simulink model "Copy_of_DSBF"  (R2019b)
settings: Solver=FixedStepDiscrete  StartTime=0.0  StopTime=stopTime  RelTol=1e-3
InitFcn:
  | initCallback
StopFcn:
  | stopCallback
values from neighbouring files (symbols this model uses):
  arraySize = mp.arraySize    [modelparameters.m]
  arraySpacing = mp.arraySpacing    [modelparameters.m]
  delayDataTypeFractionLength = mp.fractionalDelayAddrSize    [modelparameters.m]
  delayDataTypeWordLength = mp.integerDelayAddrSize + mp.fractionalDelayAddrSize    [modelparameters.m]
  mp = sm_init_avalon_signals(mp)    [sm_callback_init.m]    (also in sm_callback_stop.m = sm_stop_verify(mp))
  samplingRate = mp.samplingRate    [modelparameters.m]
  speedOfSound = mp.speedOfSound    [modelparameters.m]
  upsampleFactor = mp.upsampleFactor    [modelparameters.m]
undefined symbols (not defined in the file or in its folder): delayDataTypeSign
libraries: simulink x6, hdlsllib x4, dspsigops x2, dspmlti4 x1, dsphdlfiltering x1
settings Model: Creator=Ross  LastModifiedBy=wickh
settings SolverCC: MinimalZcImpactIntegration=on
settings DataIOCC: ReturnWorkspaceOutputs=off
settings OptimizationCC: DefaultParameterBehavior=Inlined  SimCompilerOptimization=on
settings DebuggingCC: ReadBeforeWriteMsg=DisableAll  WriteAfterWriteMsg=DisableAll  WriteAfterReadMsg=DisableAll  AlgebraicLoopMsg=error  SingleTaskRateTransMsg=error  PregeneratedLibrarySubsystemCodeDiagnostic=none  ArithmeticOperatorsInVariantConditions=warning
settings HardwareCC: ProdBitPerPointer=32  ProdBitPerSizeT=32  ProdBitPerPtrDiffT=32  ProdLargestAtomicFloat=None  ProdIntDivRoundTo=Undefined  ProdEndianess=Unspecified  ProdWordSize=32  ProdHWDeviceType=ASIC/FPGA->ASIC/FPGA  TargetBitPerPointer=64  TargetBitPerSizeT=64  TargetBitPerPtrDiffT=64  TargetLongLongMode=on  TargetIntDivRoundTo=Zero  TargetEndianess=LittleEndian  TargetWordSize=64  TargetHWDeviceType=Custom Processor->MATLAB Host Computer  ProdEqTarget=off
settings ModelReferenceCC: UpdateModelReferenceTargets=IfOutOfDate
settings SFSimCC: SFSimEcho=off  SimUseLocalCustomCode=off  CustomCodeUndefinedFunction=UseInterfaceOnly
settings RTWCC: RTWUseLocalCustomCode=off

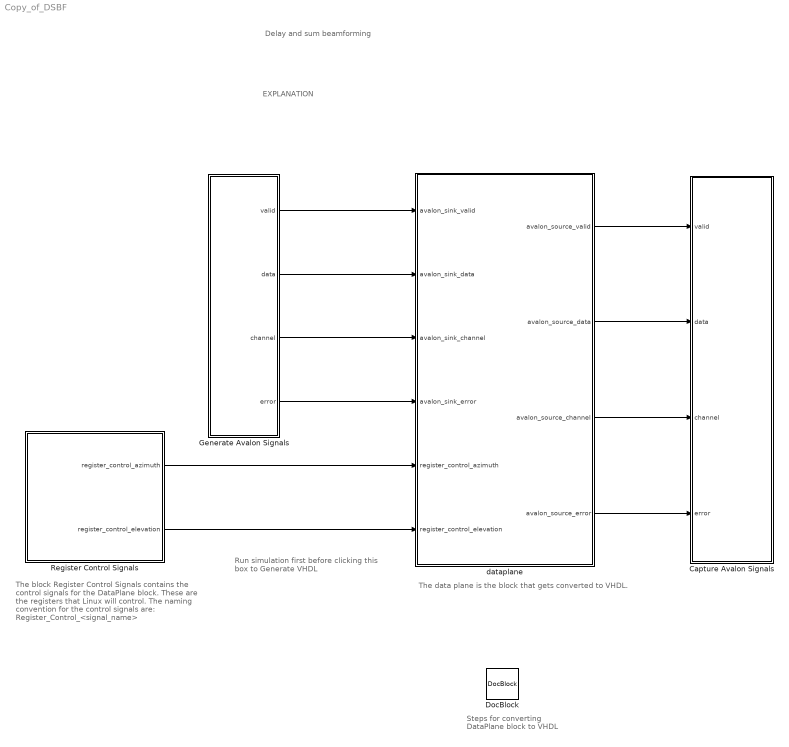
== system Copy_of_DSBF ==
  note: The data plane is the block that gets converted to VHDL.
  note: EXPLANATION
  note: Steps for converting
      | DataPlane block
      | to VHDL
  note: Delay and sum beamforming
  note: Run simulation first
      | before clicking this box to
      | Generate VHDL
  note: The block Register Control Signals contains
      | the control signals for the DataPlane block.
      | These are the registers that Linux will control.
      | The naming convention for the control
      | signals are:  Register_Control_<signal_name>
  Capture Avalon Signals : Subsystem
  DocBlock : simulink/Model-Wide Utilities/DocBlock  DocumentType=HTML
  Generate Avalon Signals : Subsystem
  Register Control Signals : Subsystem
  dataplane : Subsystem  TreatAsAtomicUnit=on
  wires:
  Generate Avalon Signals/2(data) -> dataplane/2(avalon_sink_data)
  Generate Avalon Signals/1(valid) -> dataplane/1(avalon_sink_valid)
  Generate Avalon Signals/3(channel) -> dataplane/3(avalon_sink_channel)
  Generate Avalon Signals/4(error) -> dataplane/4(avalon_sink_error)
  dataplane/2(avalon_source_data) -> Capture Avalon Signals/2(data)
  dataplane/1(avalon_source_valid) -> Capture Avalon Signals/1(valid)
  dataplane/3(avalon_source_channel) -> Capture Avalon Signals/3(channel)
  dataplane/4(avalon_source_error) -> Capture Avalon Signals/4(error)
  Register Control Signals/1(register_control_azimuth) -> dataplane/5(register_control_azimuth)
  Register Control Signals/2(register_control_elevation) -> dataplane/6(register_control_elevation)

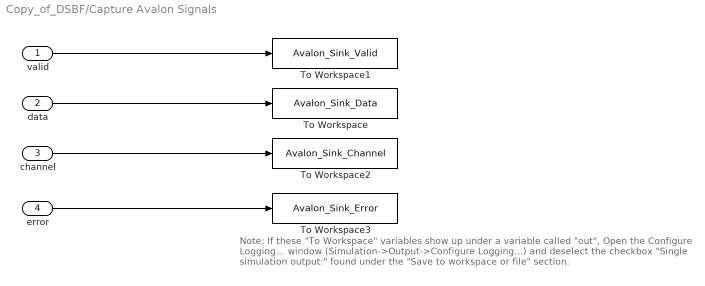
== system Copy_of_DSBF/Capture Avalon Signals ==
  note: Note:  If these "To Workspace" variables show up under a variable called "out",
      | Open the Configure Logging... window (Simulation->Output->Configure Logging...)
      | and deselect the checkbox "Single simulation output:" found under the "Save to workspace or file" section.
  valid : Inport
  data : Inport  Port=2
  channel : Inport  Port=3
  error : Inport  Port=4
  To Workspace : ToWorkspace  VariableName=Avalon_Sink_Data  SaveFormat=Timeseries  SampleTime=-1
  To Workspace1 : ToWorkspace  VariableName=Avalon_Sink_Valid  SaveFormat=Timeseries  SampleTime=-1
  To Workspace2 : ToWorkspace  VariableName=Avalon_Sink_Channel  SaveFormat=Timeseries  SampleTime=-1
  To Workspace3 : ToWorkspace  VariableName=Avalon_Sink_Error  SaveFormat=Timeseries  SampleTime=-1
  wires:
  data/1 -> To Workspace/1
  valid/1 -> To Workspace1/1
  error/1 -> To Workspace3/1
  channel/1 -> To Workspace2/1

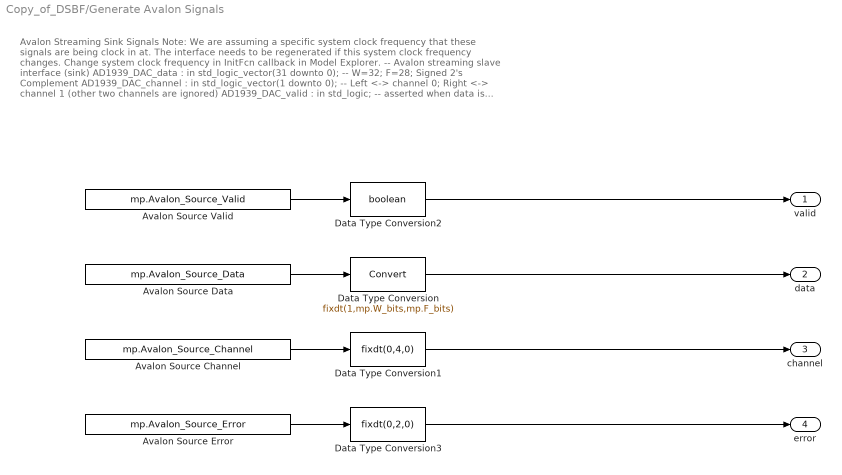
== system Copy_of_DSBF/Generate Avalon Signals ==
  note: Avalon Streaming Sink Signals
      | Note: We are assuming a specific system clock frequency that these signals are being clock in at.
      | The interface needs to be regenerated if this system clock frequency changes. Change system clock frequency in InitFcn callback in Model Explorer.
      |
      | -- Avalon streaming slave interface (sink)
      | AD1939_DAC_data : in std_logic_vector(31 downto 0); -- W=32; F=28; Signed 2's Complement
      | AD1939_DAC_channel : in std_logic_vector(1 downto 0); -- Left <-> channel 0; Right <-> channel 1 (other two channels are ignored)
      | AD1939_DAC_valid : in std_logic; -- asserted when data is valid
      | AD1939_DAC_error : in std_logic_vector(1 downto 0) -- error channel is ignored, assumed to be error free at this point
      |
      | For more information on the data-channel-valid protocol, see chapter 5 in Intel's Avalon Interfaced Specification (p. 40) at https://www.intel.com/content/dam/www/programmable/us/en/pdfs/literature/manual/mnl_avalon_spec.pdf
  Avalon Source Channel : FromWorkspace  VariableName=mp.Avalon_Source_Channel  OutDataTypeStr=double  SampleTime=mp.Ts_sim
  "Avalon Source Data " : FromWorkspace  VariableName=mp.Avalon_Source_Data  OutDataTypeStr=double  SampleTime=mp.Ts_sim
  Avalon Source Error : FromWorkspace  VariableName=mp.Avalon_Source_Error  OutDataTypeStr=double  SampleTime=mp.Ts_sim
  Avalon Source Valid : FromWorkspace  VariableName=mp.Avalon_Source_Valid  OutDataTypeStr=double  SampleTime=mp.Ts_sim
  Data Type Conversion : DataTypeConversion  OutDataTypeStr=fixdt(1,mp.W_bits,mp.F_bits)
  Data Type Conversion1 : DataTypeConversion  OutDataTypeStr=fixdt(0,4,0)
  Data Type Conversion2 : DataTypeConversion  OutDataTypeStr=boolean
  Data Type Conversion3 : DataTypeConversion  OutDataTypeStr=fixdt(0,2,0)
  valid : Outport  VectorParamsAs1DForOutWhenUnconnected=off
  data : Outport  Port=2  VectorParamsAs1DForOutWhenUnconnected=off
  channel : Outport  Port=3  VectorParamsAs1DForOutWhenUnconnected=off
  error : Outport  Port=4  VectorParamsAs1DForOutWhenUnconnected=off
  wires:
  Data Type Conversion1/1 -> channel/1
  Data Type Conversion2/1 -> valid/1
  Avalon Source Error/1 -> Data Type Conversion3/1
  Data Type Conversion/1 -> data/1
  Avalon Source Valid/1 -> Data Type Conversion2/1
  Data Type Conversion3/1 -> error/1
  Avalon Source Channel/1 -> Data Type Conversion1/1
  "Avalon Source Data "/1 -> Data Type Conversion/1

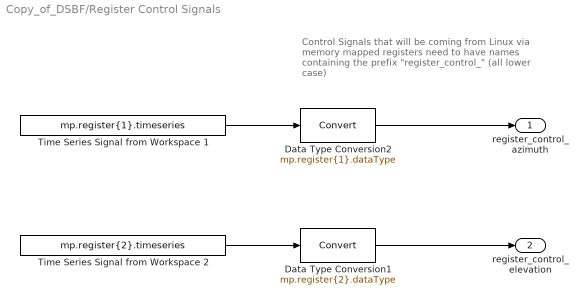
== system Copy_of_DSBF/Register Control Signals ==
  note: Control Signals that will be coming from Linux via
      | memory mapped registers need to have names
      | containing the prefix "register_control_"
      | (all lower case)
  Data Type Conversion1 : DataTypeConversion  OutDataTypeStr=mp.register{2}.dataType
  Data Type Conversion2 : DataTypeConversion  OutDataTypeStr=mp.register{1}.dataType
  Time Series Signal from Workspace 1 : FromWorkspace  VariableName=mp.register{1}.timeseries  OutDataTypeStr=double  SampleTime=mp.Ts_sim
  Time Series Signal from Workspace 2 : FromWorkspace  VariableName=mp.register{2}.timeseries  OutDataTypeStr=double  SampleTime=mp.Ts_sim
  register_control_azimuth : Outport  VectorParamsAs1DForOutWhenUnconnected=off
  register_control_elevation : Outport  Port=2  VectorParamsAs1DForOutWhenUnconnected=off
  wires:
  Time Series Signal from Workspace 1/1 -> Data Type Conversion2/1
  Time Series Signal from Workspace 2/1 -> Data Type Conversion1/1
  Data Type Conversion2/1 -> register_control_azimuth/1
  Data Type Conversion1/1 -> register_control_elevation/1

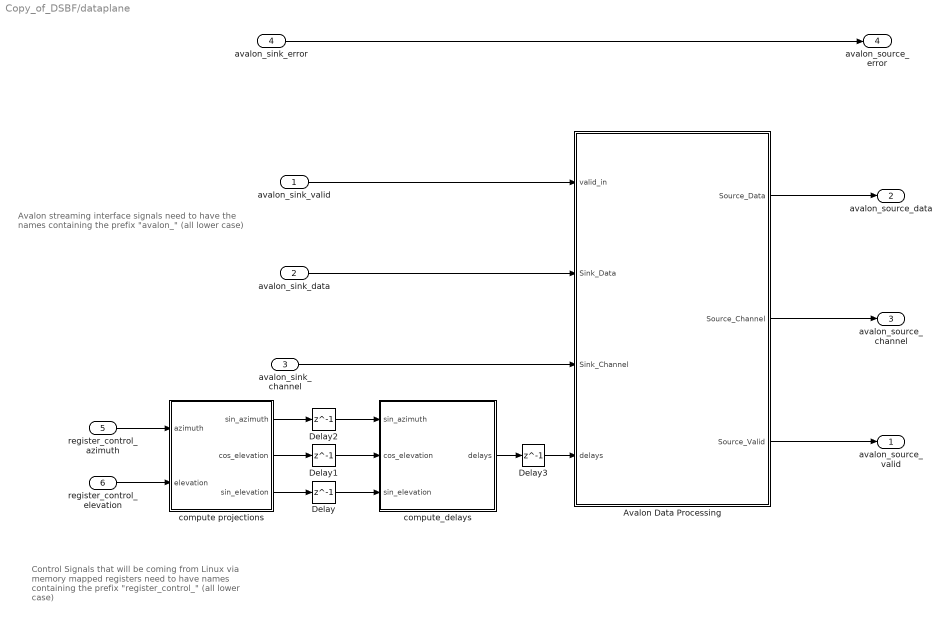
== system Copy_of_DSBF/dataplane ==
  note: Control Signals that will be coming from Linux via
      | memory mapped registers need to have names
      | containing the prefix "register_control_"
      | (all lower case)
  note: Avalon streaming interface signals need to have the
      | names containing the prefix "avalon_"
      | (all lower case)
  avalon_sink_valid : Inport
  avalon_sink_data : Inport  Port=2
  avalon_sink_channel : Inport  Port=3
  avalon_sink_error : Inport  Port=4
  register_control_azimuth : Inport  Port=5
  register_control_elevation : Inport  Port=6
  Avalon Data Processing : Subsystem  TreatAsAtomicUnit=on
  Delay{,1..3} (4 alike) : Delay  DelayLength=1
  compute projections : Subsystem
  compute_delays : MATLAB Function  TreatAsAtomicUnit=on
  avalon_source_valid : Outport  VectorParamsAs1DForOutWhenUnconnected=off
  avalon_source_data : Outport  Port=2  VectorParamsAs1DForOutWhenUnconnected=off
  avalon_source_channel : Outport  Port=3  VectorParamsAs1DForOutWhenUnconnected=off
  avalon_source_error : Outport  Port=4  VectorParamsAs1DForOutWhenUnconnected=off
  wires:
  avalon_sink_channel/1 -> Avalon Data Processing/3(Sink_Channel)
  avalon_sink_error/1 -> avalon_source_error/1
  Avalon Data Processing/1(Source_Data) -> avalon_source_data/1
  avalon_sink_data/1 -> Avalon Data Processing/2(Sink_Data)
  Avalon Data Processing/2(Source_Channel) -> avalon_source_channel/1
  compute_delays/1(delays) -> Delay3/1
  avalon_sink_valid/1 -> Avalon Data Processing/1(valid_in)
  Avalon Data Processing/3(Source_Valid) -> avalon_source_valid/1
  register_control_elevation/1 -> compute projections/2(elevation)
  register_control_azimuth/1 -> compute projections/1(azimuth)
  compute projections/1(sin_azimuth) -> Delay2/1
  compute projections/2(cos_elevation) -> Delay1/1
  compute projections/3(sin_elevation) -> Delay/1
  Delay/1 -> compute_delays/3(sin_elevation)
  Delay1/1 -> compute_delays/2(cos_elevation)
  Delay2/1 -> compute_delays/1(sin_azimuth)
  Delay3/1 -> Avalon Data Processing/4(delays)

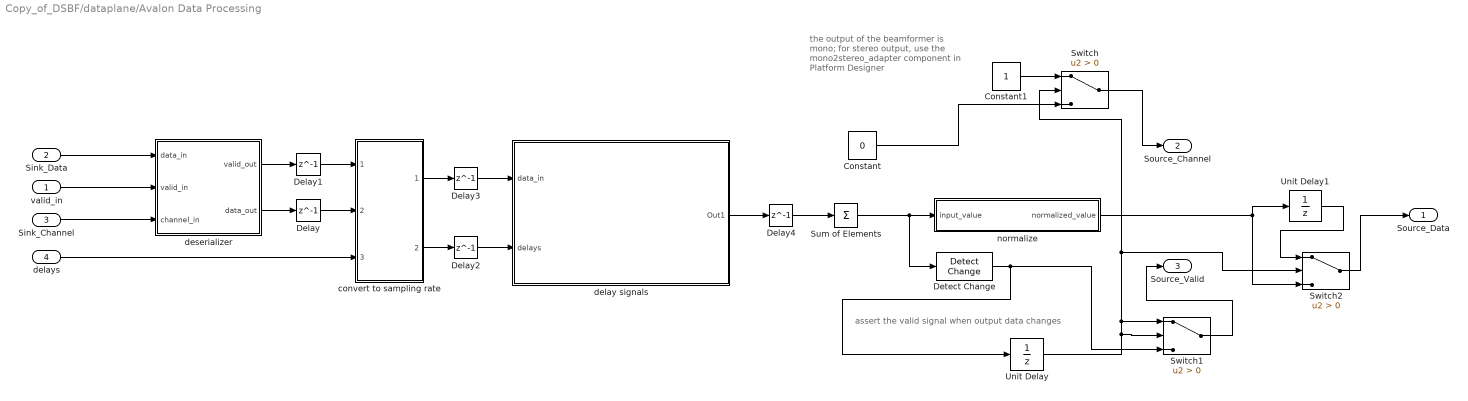
== system Copy_of_DSBF/dataplane/Avalon Data Processing ==
  note: assert the valid signal when output data changes
  note: the output of the beamformer is mono; for stereo output, use the mono2stereo_adapter component in Platform Designer
  valid_in : Inport
  Sink_Data : Inport  Port=2
  Sink_Channel : Inport  Port=3
  delays : Inport  Port=4
  Constant : Constant  Value=0  OutDataTypeStr=fixdt(0,1,0)  SampleTime=-1
  Constant1 : Constant  OutDataTypeStr=fixdt(0,1)  SampleTime=-1
  Delay{,1..4} (5 alike) : Delay  DelayLength=1
  Detect Change : simulink/Logic and Bit Operations/Detect Change  vinit=0  OutDataTypeStr=boolean
  Sum of Elements : Sum  Inputs=+  CollapseMode=Specified dimension
  Switch : Switch  Criteria=u2 > Threshold
  Switch1 : Switch  Criteria=u2 > Threshold
  Switch2 : Switch  Criteria=u2 > Threshold
  Unit Delay : UnitDelay  SampleTime=-1  HasFrameUpgradeWarning=on
  Unit Delay1 : UnitDelay  SampleTime=-1  HasFrameUpgradeWarning=on
  convert to sampling rate : Subsystem
  delay signals : Subsystem  TreatAsAtomicUnit=on
  deserializer : MATLAB Function  TreatAsAtomicUnit=on
  normalize : Subsystem
  Source_Data : Outport  InitialOutput=0  VectorParamsAs1DForOutWhenUnconnected=off
  Source_Channel : Outport  Port=2  InitialOutput=0  VectorParamsAs1DForOutWhenUnconnected=off
  Source_Valid : Outport  Port=3  InitialOutput=0  VectorParamsAs1DForOutWhenUnconnected=off
  wires:
  valid_in/1 -> deserializer/2(valid_in)
  Sink_Data/1 -> deserializer/1(data_in)
  delays/1 -> convert to sampling rate/3(delays_in)
  Sink_Channel/1 -> deserializer/3(channel_in)
  Sum of Elements/1 -> Detect Change/1, normalize/1(input_value)
  Constant/1 -> Switch/3
  convert to sampling rate/2(delays_out) -> Delay2/1
  convert to sampling rate/1(data_out) -> Delay3/1
  deserializer/2(data_out) -> Delay/1
  deserializer/1(valid_out) -> Delay1/1
  delay signals/1(Out1) -> Delay4/1
  Detect Change/1 -> Unit Delay/1, Switch1/3
  normalize/1(normalized_value) -> Switch2/3, Unit Delay1/1
  Delay/1 -> convert to sampling rate/2(data_in)
  Delay1/1 -> convert to sampling rate/1(valid_in)
  Delay2/1 -> delay signals/2(delays)
  Delay3/1 -> delay signals/1(data_in)
  Delay4/1 -> Sum of Elements/1
  Unit Delay/1 -> Switch1/2, Switch1/1, Switch2/2, Switch/2
  Switch/1 -> Source_Channel/1
  Switch1/1 -> Source_Valid/1
  Unit Delay1/1 -> Switch2/1
  Switch2/1 -> Source_Data/1
  Constant1/1 -> Switch/1

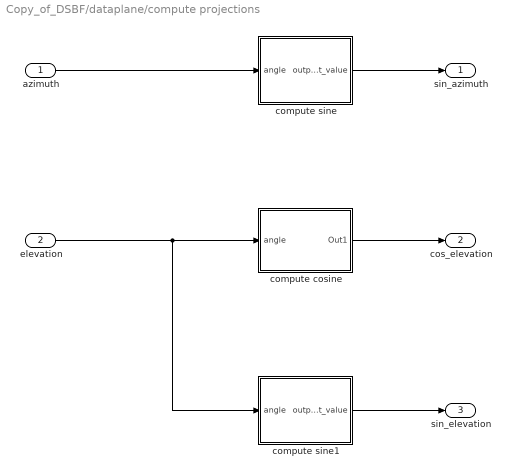
== system Copy_of_DSBF/dataplane/compute projections ==
  azimuth : Inport
  elevation : Inport  Port=2
  compute cosine : Subsystem
  compute sine : Subsystem
  compute sine1 : Subsystem
  sin_azimuth : Outport
  cos_elevation : Outport  Port=2
  sin_elevation : Outport  Port=3
  wires:
  elevation/1 -> compute sine1/1(angle), compute cosine/1(angle)
  azimuth/1 -> compute sine/1(angle)
  compute sine1/1(output_value) -> sin_elevation/1
  compute cosine/1(Out1) -> cos_elevation/1
  compute sine/1(output_value) -> sin_azimuth/1

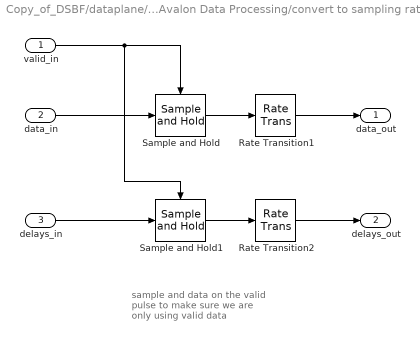
== system Copy_of_DSBF/dataplane/Avalon Data Processing/convert to sampling rate ==
  note: sample and data on the valid pulse to make sure we are only using valid data
  valid_in : Inport
  data_in : Inport  Port=2
  delays_in : Inport  Port=3
  Rate Transition1 : RateTransition  OutPortSampleTime=mp.Ts
  Rate Transition2 : RateTransition  OutPortSampleTime=mp.Ts
  Sample and Hold : dspsigops/Sample and Hold  trig=Rising edge  initCond=0  latchinput=off
  Sample and Hold1 : dspsigops/Sample and Hold  trig=Rising edge  initCond=0  latchinput=off
  data_out : Outport
  delays_out : Outport  Port=2
  wires:
  Sample and Hold/1 -> Rate Transition1/1
  data_in/1 -> Sample and Hold/1
  Rate Transition1/1 -> data_out/1
  valid_in/1 -> Sample and Hold1/Trigger, Sample and Hold/Trigger
  delays_in/1 -> Sample and Hold1/1
  Sample and Hold1/1 -> Rate Transition2/1
  Rate Transition2/1 -> delays_out/1

== system Copy_of_DSBF/dataplane/Avalon Data Processing/delay signals ==
  data_in : Inport  Partition=on  PartitionDimension=1  PartitionWidth=1  PartitionOffset=0
  delays : Inport  Port=2  Partition=on  PartitionDimension=1  PartitionWidth=1  PartitionOffset=0
  For Each : ForEach  DisableCoverage=on
  delay signal : Subsystem
  Out1 : Outport  ConcatenationDimension=1  VectorParamsAs1DForOutWhenUnconnected=off
  wires:
  delay signal/1(data_out) -> Out1/1
  data_in/1 -> delay signal/1(data_in)
  delays/1 -> delay signal/2(delay)

== system Copy_of_DSBF/dataplane/Avalon Data Processing/normalize ==
  input_value : Inport
  Data Type Conversion : DataTypeConversion  OutDataTypeStr=fixdt(1, mp.W_bits, mp.F_bits)
  normalize_shift : MATLAB Function  TreatAsAtomicUnit=on
  normalized_value : Outport
  wires:
  input_value/1 -> normalize_shift/1(input)
  Data Type Conversion/1 -> normalized_value/1
  normalize_shift/1(normalized) -> Data Type Conversion/1

== system Copy_of_DSBF/dataplane/compute projections/compute cosine ==
  note: cosine has even symmetry on [-90, 90].
      | we can take advantage of that and only compute values on [0 90]
  angle : Inport
  Abs : Abs
  cos LUT : Subsystem  Description=This block was created using function approximation.
  Out1 : Outport
  wires:
  cos LUT/1(Out1) -> Out1/1
  angle/1 -> Abs/1
  Abs/1 -> cos LUT/1(In1)

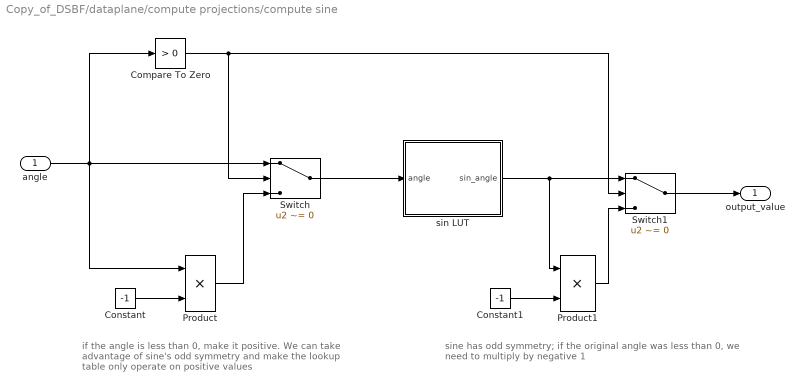
== system Copy_of_DSBF/dataplane/compute projections/compute sine ==
  note: if the angle is less than 0, make it positive.
      | We can take advantage of sine's odd symmetry and
      | make the lookup table only operate on positive values
  note: sine has odd symmetry; if the original angle was less than 0,
      | we need to multiply by negative 1
  angle : Inport
  Compare To Zero : simulink/Logic and Bit Operations/Compare To Zero  relop=>  OutDataTypeStr=boolean
  Constant : Constant  Value=-1  OutDataTypeStr=Inherit: Inherit via back propagation  SampleTime=-1
  Constant1 : Constant  Value=-1  OutDataTypeStr=Inherit: Inherit via back propagation  SampleTime=-1
  Product : Product  OutDataTypeStr=Inherit: Same as first input
  Product1 : Product  OutDataTypeStr=Inherit: Same as first input
  Switch : Switch  Criteria=u2 ~= 0  Threshold=1
  Switch1 : Switch  Criteria=u2 ~= 0  Threshold=1
  sin LUT : Subsystem  Description=This block was created using function approximation.
  output_value : Outport
  wires:
  Switch/1 -> sin LUT/1(angle)
  Constant/1 -> Product/2
  angle/1 -> Compare To Zero/1, Product/1, Switch/1
  Constant1/1 -> Product1/2
  Switch1/1 -> output_value/1
  sin LUT/1(sin_angle) -> Product1/1, Switch1/1
  Compare To Zero/1 -> Switch/2, Switch1/2
  Product1/1 -> Switch1/3
  Product/1 -> Switch/3

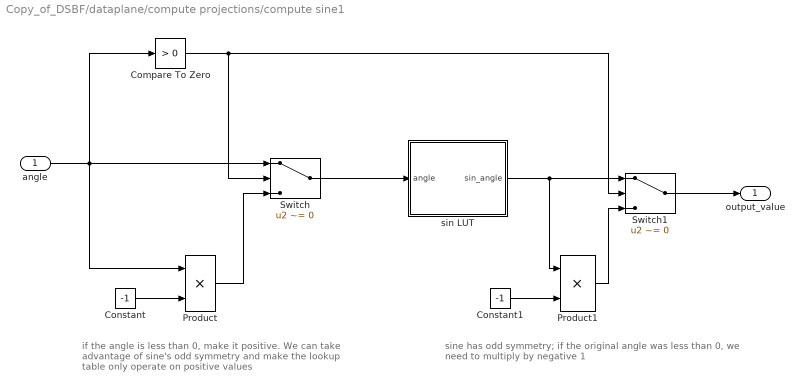
== system Copy_of_DSBF/dataplane/compute projections/compute sine1 ==
  note: if the angle is less than 0, make it positive.
      | We can take advantage of sine's odd symmetry and
      | make the lookup table only operate on positive values
  note: sine has odd symmetry; if the original angle was less than 0,
      | we need to multiply by negative 1
  angle : Inport
  Compare To Zero : simulink/Logic and Bit Operations/Compare To Zero  relop=>  OutDataTypeStr=boolean
  Constant : Constant  Value=-1  OutDataTypeStr=Inherit: Inherit via back propagation  SampleTime=-1
  Constant1 : Constant  Value=-1  OutDataTypeStr=Inherit: Inherit via back propagation  SampleTime=-1
  Product : Product  OutDataTypeStr=Inherit: Same as first input
  Product1 : Product  OutDataTypeStr=Inherit: Same as first input
  Switch : Switch  Criteria=u2 ~= 0  Threshold=1
  Switch1 : Switch  Criteria=u2 ~= 0  Threshold=1
  sin LUT : Subsystem  Description=This block was created using function approximation.
  output_value : Outport
  wires:
  Switch/1 -> sin LUT/1(angle)
  Constant/1 -> Product/2
  angle/1 -> Compare To Zero/1, Product/1, Switch/1
  Constant1/1 -> Product1/2
  Switch1/1 -> output_value/1
  sin LUT/1(sin_angle) -> Product1/1, Switch1/1
  Compare To Zero/1 -> Switch/2, Switch1/2
  Product1/1 -> Switch1/3
  Product/1 -> Switch/3

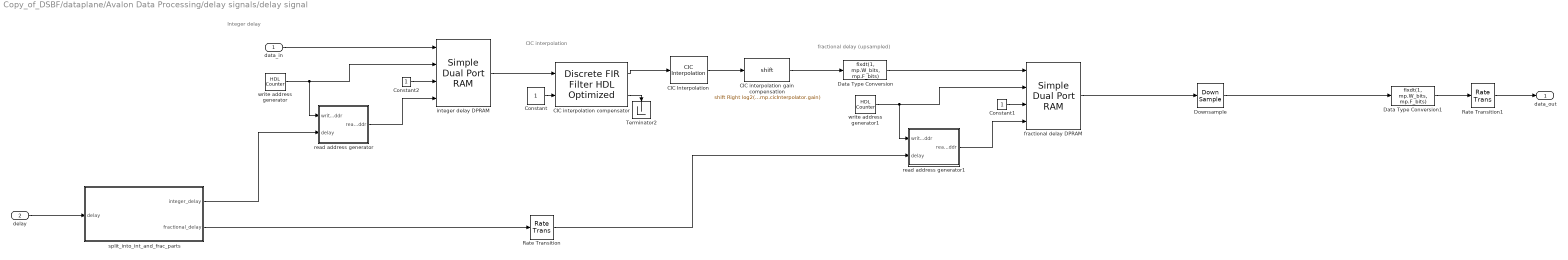
== system Copy_of_DSBF/dataplane/Avalon Data Processing/delay signals/delay signal ==
  note: CIC interpolation
  note: Integer delay
  note: fractional delay (upsampled)
  data_in : Inport
  delay : Inport  Port=2
  CIC Interpolation : dspmlti4/CIC Interpolation  filtFrom=Filter object  filtobj=mp.cicInterpolator  ftype=Interpolator  R=mp.upsampleFactor  M=1  N=2  filterInternals=Full precision  BPS=[16 16 16 16]  FLPS=0  outputWordLength=32  outputFracLength=0  launchFVT=off  framing=Allow multirate processing  OutputFrames=off
      settings: SourceProductName=DSP System Toolbox  SourceProductBaseCode=DS
  CIC interpolation compensator : dsphdlfiltering/Discrete FIR Filter HDL Optimized  NumeratorSource=Property  Numerator=mp.cicInterpolatorCompensator.coeffs.Numerator  NumeratorPrototype=[]  FilterStructure=Direct form systolic  SerializationOption=Maximum number of multipliers  NumberOfCycles=2  NumberOfMultipliers=4  SimulateUsing=Code generation  roundingMode=Floor  overflowMode=off  CoefficientsDataTypeStr=fixdt(1,16)  CoefficientsMin=[]  CoefficientsMax=[]  OutputDataTypeStr=Inherit: Same word length as input  OutputMin=[]  OutputMax=[]  ResetInputPort=off  HDLGlobalReset=off
      settings: SourceProductName=DSP System Toolbox  SourceProductBaseCode=DS
  CIC interpolation gain compensation : ArithShift  BitShiftNumber=log2(mp.cicInterpolator.gain)  BitShiftDirection=Right  DiagnosticForOORShift=Error
  Constant : Constant  OutDataTypeStr=boolean  SampleTime=-1
  Constant1 : Constant  OutDataTypeStr=Inherit: Inherit via back propagation  SampleTime=-1
  Constant2 : Constant  OutDataTypeStr=Inherit: Inherit via back propagation  SampleTime=-1
  Data Type Conversion : DataTypeConversion  OutDataTypeStr=fixdt(1, mp.W_bits, mp.F_bits)
  Data Type Conversion1 : DataTypeConversion  OutDataTypeStr=fixdt(1, mp.W_bits, mp.F_bits)
  Downsample : DownSample  N=mp.upsampleFactor  RateOptions=Allow multirate processing
  Rate Transition : RateTransition  OutPortSampleTime=mp.Ts/mp.upsampleFactor
  Rate Transition1 : RateTransition  OutPortSampleTime=mp.Ts_sim
  Terminator2 : Terminator
  fractional delay DPRAM : hdlsllib/HDL RAMs/Simple Dual Port RAM  ram_size=mp.fractionalDelayAddrSize
      settings: SourceProductName=Simulink  SourceProductBaseCode=SL
  integer delay DPRAM : hdlsllib/HDL RAMs/Simple Dual Port RAM  ram_size=mp.integerDelayAddrSize
      settings: SourceProductName=Simulink  SourceProductBaseCode=SL
  read address generator : Subsystem
  read address generator1 : Subsystem
  split_into_int_and_frac_parts : MATLAB Function  TreatAsAtomicUnit=on
  write address generator : hdlsllib/Sources/HDL Counter  CountType=Count limited  CountInit=0  CountStep=1  CountMax=mp.integerDelayBufferSize - 1  CountFromType=Initial value  CountFrom=0  CountResetPort=off  CountLoadPort=off  CountEnbPort=off  CountDirPort=off  CountDataType=Unsigned  CountWordLen=mp.integerDelayAddrSize  CountFracLen=0  CountSampTime=-1
      settings: SourceProductName=Simulink
  write address generator1 : hdlsllib/Sources/HDL Counter  CountType=Count limited  CountInit=0  CountStep=1  CountMax=mp.fractionalDelayBufferSize - 1  CountFromType=Initial value  CountFrom=0  CountResetPort=off  CountLoadPort=off  CountEnbPort=off  CountDirPort=off  CountDataType=Unsigned  CountWordLen=mp.fractionalDelayAddrSize  CountFracLen=0  CountSampTime=-1
      settings: SourceProductName=Simulink
  data_out : Outport  VectorParamsAs1DForOutWhenUnconnected=off
  wires:
  data_in/1 -> integer delay DPRAM/1
  read address generator/1(read_addr) -> integer delay DPRAM/4
  write address generator/1 -> integer delay DPRAM/2, read address generator/1(write_addr)
  write address generator1/1 -> fractional delay DPRAM/2, read address generator1/1(write_addr)
  Constant1/1 -> fractional delay DPRAM/3
  read address generator1/1(read_addr) -> fractional delay DPRAM/4
  Constant2/1 -> integer delay DPRAM/3
  Rate Transition/1 -> read address generator1/2(delay)
  Rate Transition1/1 -> data_out/1
  Data Type Conversion/1 -> fractional delay DPRAM/1
  delay/1 -> split_into_int_and_frac_parts/1(delay)
  split_into_int_and_frac_parts/2(fractional_delay) -> Rate Transition/1
  split_into_int_and_frac_parts/1(integer_delay) -> read address generator/2(delay)
  Data Type Conversion1/1 -> Rate Transition1/1
  CIC interpolation compensator/1 -> CIC Interpolation/1
  integer delay DPRAM/1 -> CIC interpolation compensator/1
  CIC interpolation compensator/2 -> Terminator2/1
  Constant/1 -> CIC interpolation compensator/2
  CIC Interpolation/1 -> CIC interpolation gain compensation/1
  CIC interpolation gain compensation/1 -> Data Type Conversion/1
  fractional delay DPRAM/1 -> Downsample/1
  Downsample/1 -> Data Type Conversion1/1

== system Copy_of_DSBF/dataplane/compute projections/compute cosine/cos LUT ==
  In1 : Inport
  DTC1 : DataTypeConversion  RndMeth=Nearest
  LUT : Lookup_n-D  NumberOfTableDimensions=1  LookupTableObject=FunctionApproximation_LUTObject_20200313T090826873  BreakpointsSpecification=Even spacing  BreakpointsForDimension3=[5, 7]  BreakpointsForDimension1FirstPoint=0  BreakpointsForDimension1Spacing=2  IndexSearchMethod=Evenly spaced points  BeginIndexSearchUsingPreviousIndexResult=on  Table=[1 0.9993896484375 0.99755859375 0.9945068359375 0.99029541015625 0.98480224609375 0.9781494140625 0.97027587890625 0.96124267578125 0.9510498046875 0.939697265625 0.92718505859375 0.91357421875 0.8988037109375 0.8829345703125 0.86602783203125 0.8480224609375 0.82904052734375 0.80902099609375 0.78802490234375 0.76605224609375 0.7431640625 0.7193603515625 0.69464111328125 0.66912841796875 0.64276123046875 0.61566162109375 0.5877685546875 0.5592041015625 0.5299072265625 0.5 0.469482421875 0.4383544921875 0.40673828125 0.3746337890625 0.342041015625 0.30902099609375 0.275634765625 0.241943359375 0.2078857421875 0.17364501953125 0.13916015625 0.10455322265625 0.06976318359375 0.034912109375 0]  TableDataTypeStr=numerictype(1,16,14)  ExtrapMethod=Clip  DiagnosticForOutOfRangeInput=Error  UseLastTableValue=on  InternalRulePriority=Speed  OutDataTypeStr=numerictype(1,16,14)  RndMeth=Simplest
  SigSpec1 : SignalSpecification  OutMin=0  OutMax=90  OutDataTypeStr=numerictype(1,16,8)
  Out1 : Outport
  wires:
  LUT/1 -> Out1/1
  In1/1 -> DTC1/1
  SigSpec1/1 -> LUT/1
  DTC1/1 -> SigSpec1/1

== system Copy_of_DSBF/dataplane/compute projections/compute sine/sin LUT ==
  angle : Inport
  DTC2 : DataTypeConversion  RndMeth=Nearest
  LUT1 : Lookup_n-D  NumberOfTableDimensions=1  LookupTableObject=FunctionApproximation_LUTObject_20200313T084211896  BreakpointsSpecification=Even spacing  BreakpointsForDimension3=[5, 7]  BreakpointsForDimension1FirstPoint=0  BreakpointsForDimension1Spacing=4  IndexSearchMethod=Evenly spaced points  BeginIndexSearchUsingPreviousIndexResult=on  Table=[0 0.06976318359375 0.13916015625 0.2078857421875 0.275634765625 0.342041015625 0.40673828125 0.469482421875 0.5299072265625 0.5877685546875 0.64276123046875 0.69464111328125 0.7431640625 0.78802490234375 0.82904052734375 0.86602783203125 0.8988037109375 0.92718505859375 0.9510498046875 0.97027587890625 0.98480224609375 0.9945068359375 0.9993896484375]  TableDataTypeStr=numerictype(1,16,14)  ExtrapMethod=Clip  DiagnosticForOutOfRangeInput=Error  UseLastTableValue=on  InternalRulePriority=Speed  OutDataTypeStr=numerictype(1,16,14)  RndMeth=Simplest
  SigSpec2 : SignalSpecification  OutMin=0  OutMax=90  OutDataTypeStr=numerictype(1,16,8)
  sin_angle : Outport
  wires:
  SigSpec2/1 -> LUT1/1
  LUT1/1 -> sin_angle/1
  DTC2/1 -> SigSpec2/1
  angle/1 -> DTC2/1

== system Copy_of_DSBF/dataplane/compute projections/compute sine1/sin LUT ==
  angle : Inport
  DTC2 : DataTypeConversion  RndMeth=Nearest
  LUT1 : Lookup_n-D  NumberOfTableDimensions=1  LookupTableObject=FunctionApproximation_LUTObject_20200313T084211896  BreakpointsSpecification=Even spacing  BreakpointsForDimension3=[5, 7]  BreakpointsForDimension1FirstPoint=0  BreakpointsForDimension1Spacing=4  IndexSearchMethod=Evenly spaced points  BeginIndexSearchUsingPreviousIndexResult=on  Table=[0 0.06976318359375 0.13916015625 0.2078857421875 0.275634765625 0.342041015625 0.40673828125 0.469482421875 0.5299072265625 0.5877685546875 0.64276123046875 0.69464111328125 0.7431640625 0.78802490234375 0.82904052734375 0.86602783203125 0.8988037109375 0.92718505859375 0.9510498046875 0.97027587890625 0.98480224609375 0.9945068359375 0.9993896484375]  TableDataTypeStr=numerictype(1,16,14)  ExtrapMethod=Clip  DiagnosticForOutOfRangeInput=Error  UseLastTableValue=on  InternalRulePriority=Speed  OutDataTypeStr=numerictype(1,16,14)  RndMeth=Simplest
  SigSpec2 : SignalSpecification  OutMin=0  OutMax=90  OutDataTypeStr=numerictype(1,16,8)
  sin_angle : Outport
  wires:
  SigSpec2/1 -> LUT1/1
  LUT1/1 -> sin_angle/1
  DTC2/1 -> SigSpec2/1
  angle/1 -> DTC2/1

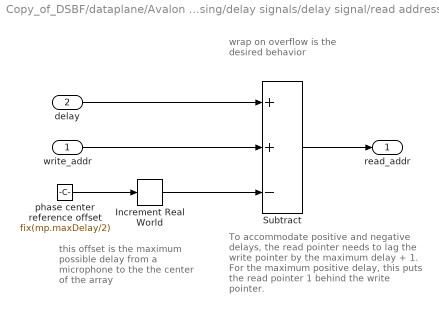
== system Copy_of_DSBF/dataplane/Avalon Data Processing/delay signals/delay signal/read address generator ==
  note: To accommodate positive and negative delays, the read pointer needs to lag the write pointer by the maximum delay + 1. For the maximum positive delay, this puts the read pointer 1 behind the write pointer.
  note: this offset is the maximum possible delay from a microphone to the the center of the array
  note: wrap on overflow is the desired behavior
  write_addr : Inport
  delay : Inport  Port=2
  Increment Real World : simulink/Additional Math & Discrete/Additional Math: Increment - Decrement/Increment Real World
      settings: SourceProductName=Simulink  SourceProductBaseCode=SL
  Subtract : Sum  Inputs=++-  OutDataTypeStr=Inherit: Inherit via back propagation
  phase center reference offset : Constant  Value=fix(mp.maxDelay/2)  OutDataTypeStr=fixdt(0,delayDataTypeWordLength - delayDataTypeFractionLength,0)  SampleTime=-1
  read_addr : Outport  VectorParamsAs1DForOutWhenUnconnected=off
  wires:
  delay/1 -> Subtract/1
  write_addr/1 -> Subtract/2
  phase center reference offset/1 -> Increment Real World/1
  Increment Real World/1 -> Subtract/3
  Subtract/1 -> read_addr/1

== system Copy_of_DSBF/dataplane/Avalon Data Processing/delay signals/delay signal/read address generator1 ==
  note: wrap on overflow is the desired behavior
  note: To accommodate positive and negative delays, the read pointer needs to lag the write pointer by the maximum delay + 1. For the maximum positive delay, this puts the read pointer 1 behind the write pointer.
  note: this offset is the maximum possible delay from a microphone to the the center of the array
  write_addr : Inport
  delay : Inport  Port=2
  Increment Real World : simulink/Additional Math & Discrete/Additional Math: Increment - Decrement/Increment Real World
      settings: SourceProductName=Simulink  SourceProductBaseCode=SL
  Subtract : Sum  Inputs=++-  OutDataTypeStr=Inherit: Inherit via back propagation
  phase center reference offset : Constant  Value=fix(mp.upsampleFactor)  OutDataTypeStr=fixdt(0, delayDataTypeFractionLength, 0)  SampleTime=-1
  read_addr : Outport  VectorParamsAs1DForOutWhenUnconnected=off
  wires:
  delay/1 -> Subtract/1
  write_addr/1 -> Subtract/2
  phase center reference offset/1 -> Increment Real World/1
  Increment Real World/1 -> Subtract/3
  Subtract/1 -> read_addr/1

== matlab function Copy_of_DSBF/dataplane/Avalon Data Processing/deserializer ==
  data: valid_out output; data_in input; data_out output; valid_in input; channel_in input; arraySize parameter
function [valid_out, data_out] = deserialize(data_in, valid_in, channel_in, arraySize)
%#codegen
persistent data_out_temp
persistent data_out_reg

if isempty(data_out_temp)
    data_out_temp = fi(zeros(arraySize(1)*arraySize(2), 1), data_in.numerictype);
end
if isempty(data_out_reg)
    data_out_reg = fi(zeros(arraySize(1)*arraySize(2), 1), data_in.numerictype);
end

valid_out = false;
data_out = data_out_reg;


if valid_in
    data_out_temp(channel_in + 1) = data_in;
    if channel_in == length(data_out_temp) - 1
        valid_out = true;
        data_out_reg = data_out_temp;
    end
else
end

== matlab function Copy_of_DSBF/dataplane/compute_delays ==
  data: sin_azimuth input; delays output; cos_elevation input; sin_elevation input; delayDataTypeSign parameter; delayDataTypeWordLength parameter; delayDataTypeFractionLength parameter; arraySize parameter; arraySpacing parameter; speedOfSound parameter; samplingRate parameter
function delays = computeDelays(sin_azimuth, cos_elevation, sin_elevation, delayDataTypeSign, delayDataTypeWordLength, delayDataTypeFractionLength, ...
    arraySize, arraySpacing, speedOfSound, samplingRate)
%#codegen    
ELEMENT_SPACING = fi(arraySpacing, 0, 16, 15);  % meters
SPEED_OF_SOUND = fi(speedOfSound, 0, 9, 0); % meters/second
NUM_ELEMENTS_Y = fi(arraySize(1), 1, 5, 1);
NUM_ELEMENTS_Z = fi(arraySize(2), 1, 5, 1);
SAMPLING_RATE = sfi(samplingRate);

delays = fi(zeros(arraySize(1) * arraySize(2), 1), delayDataTypeSign, delayDataTypeWordLength, delayDataTypeFractionLength);
yElementIdx = fi(0:(NUM_ELEMENTS_Y - 1), 1, 5, 1);
zElementIdx = fi((0:(NUM_ELEMENTS_Z - 1)), 1, 5, 1);

yDistanceFromPhaseCenter = ELEMENT_SPACING * (yElementIdx - (NUM_ELEMENTS_Y - 1)/2);
zDistanceFromPhaseCenter = ELEMENT_SPACING * (zElementIdx - (NUM_ELEMENTS_Z - 1)/2);

idx = fi(0, 0, log2(arraySize(1) * arraySize(2)) + 1, 0, 'SumMode', 'SpecifyPrecision', ...
    'SumWordLength', log2(arraySize(1) * arraySize(2)) + 1, 'SumFractionLength', 0);
for z = zElementIdx
    for y = yElementIdx
        idx = idx + 1;
        delays(idx) = -SAMPLING_RATE/SPEED_OF_SOUND  * (yDistanceFromPhaseCenter(y + 1) * sin_azimuth * cos_elevation + ...
            zDistanceFromPhaseCenter(z + 1) * sin_elevation);
    end
end
end

== matlab function Copy_of_DSBF/dataplane/Avalon Data Processing/delay signals/delay signal/split_into_int_and_frac_parts ==
  data: delay input; integer_delay output; fractional_delay output; upsampleFactor parameter; delayDataTypeFractionLength parameter
function [integer_delay, fractional_delay] = split_delay_into_int_and_frac_parts(delay, upsampleFactor, delayDataTypeFractionLength)
%#codegen
% truncate the delay value to get the integer part
integer_delay = fix(delay);

% get the fractional part of the delay and
% convert it to an integer at the upsampled clock rate
fractional_delay_temp = delay - integer_delay;
fractional_delay_temp_upsampled = round(upsampleFactor * fractional_delay_temp);
fractional_delay = fi(fractional_delay_temp_upsampled, 1, delayDataTypeFractionLength, 0);
end

== matlab function Copy_of_DSBF/dataplane/Avalon Data Processing/normalize/normalize_shift ==
  data: input input; normalized output
function normalized = fcn(input)
%#codegen
% NOTE: we should be normalizing to +/- 1 with the following commented line,
% but the AD1939 VHDL expects +/- 0.5 normalization; so for now, I'm 
% normalizing to +/- 0.5 until we fix the VHDL
%excessIntegerBits = input.WordLength - input.FractionLength - 1;
excessIntegerBits = input.WordLength - input.FractionLength;
normalized = bitsra(input, excessIntegerBits);
end
